simulink model "mass_model"  (R2023a)
settings: Solver=FixedStepAuto  StartTime=0.0  StopTime=10.0  FixedStep=0.4  RelTol=1e-3
libraries: simulink x2, rllib x1
settings Model: Creator=mori_keigo  LastModifiedBy=mori_keigo
settings OptimizationCC: ReuseModelBlockBuffer=off

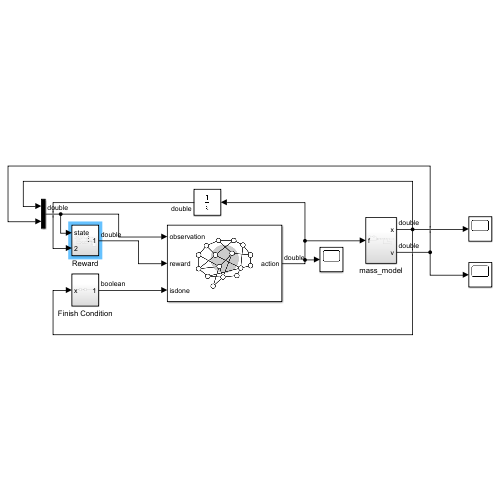
[thumbnail: Simulink's stored preview of the top-level diagram]
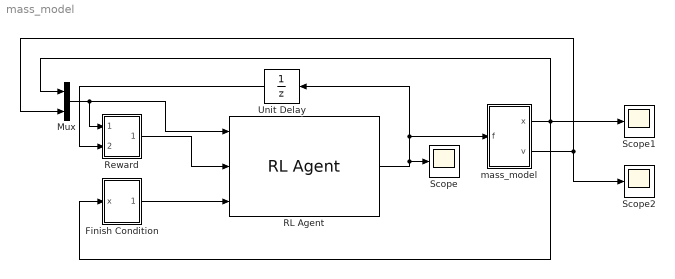
== system mass_model ==
  Finish Condition : Subsystem
  Mux : Mux  Inputs=2
  RL Agent : rllib/RL Agent  Agent=agentObj  ExternalActionAsInput=off  ProvideLastAction=off  ProvideCumRwd=off  TreatAsDirectFeedthrough=on  UseStrictObservationDataTypes=off
  Reward : Subsystem
  Scope : Scope
  Scope1 : Scope
  Scope2 : Scope
  Unit Delay : UnitDelay  SampleTime=-1  HasFrameUpgradeWarning=on
  mass_model : Subsystem
  wires:
  RL Agent/1 -> Unit Delay/1, mass_model/1(f), Scope/1
  mass_model/1(x) -> Scope1/1, Mux/1, Finish Condition/1(x)
  mass_model/2(v) -> Scope2/1, Mux/2
  Mux/1 -> Reward/1(state), RL Agent/1
  Reward/1(Out1) -> RL Agent/2
  Finish Condition/1(Out1) -> RL Agent/3
  Unit Delay/1 -> Reward/2(In2)

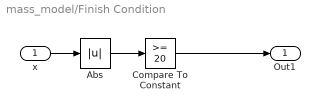
== system mass_model/Finish Condition ==
  x : Inport
  Abs : Abs  SaturateOnIntegerOverflow=off
  Compare To Constant : simulink/Logic and Bit Operations/Compare To Constant  relop=>=  const=20  OutDataTypeStr=boolean
  Out1 : Outport
  wires:
  Compare To Constant/1 -> Out1/1
  Abs/1 -> Compare To Constant/1
  x/1 -> Abs/1

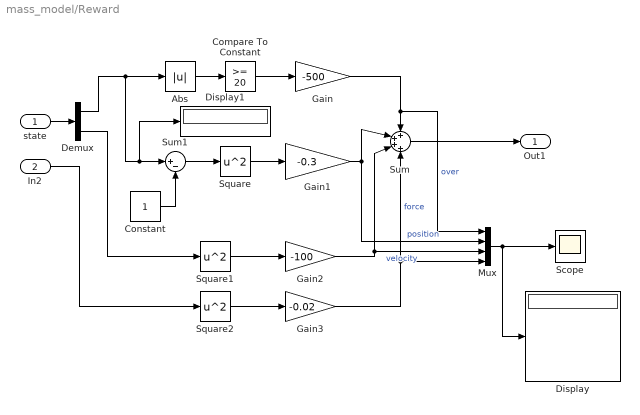
== system mass_model/Reward ==
  state : Inport
  In2 : Inport  Port=2
  Abs : Abs  SaturateOnIntegerOverflow=off
  Compare To Constant : simulink/Logic and Bit Operations/Compare To Constant  relop=>=  const=20  OutDataTypeStr=boolean
  Constant : Constant
  Demux : Demux  Outputs=2
  Display : Display
  Display1 : Display
  Gain : Gain  Gain=-500  OutDataTypeStr=double
  Gain1 : Gain  Gain=-0.3
  Gain2 : Gain  Gain=-100
  Gain3 : Gain  Gain=-0.02
  Mux : Mux
  Scope : Scope
  Square : Math  Operator=square
  Square1 : Math  Operator=square
  Square2 : Math  Operator=square
  Sum : Sum  Inputs=++++
  Sum1 : Sum  Inputs=|+-
  Out1 : Outport
  wires:
  state/1 -> Demux/1
  Demux/1 -> Display1/1, Sum1/1, Abs/1
  Abs/1 -> Compare To Constant/1
  Compare To Constant/1 -> Gain/1
  Square/1 -> Gain1/1
  Square1/1 -> Gain2/1
  Demux/2 -> Square1/1
  Gain/1 -> Mux/1, Sum/1  "over"
  Gain1/1 -> Mux/2, Sum/2  "position"
  Gain2/1 -> Mux/3, Sum/3  "velocity"
  Sum/1 -> Out1/1
  Constant/1 -> Sum1/2
  Sum1/1 -> Square/1
  In2/1 -> Square2/1
  Square2/1 -> Gain3/1
  Gain3/1 -> Mux/4, Sum/4  "force"
  Mux/1 -> Display/1, Scope/1

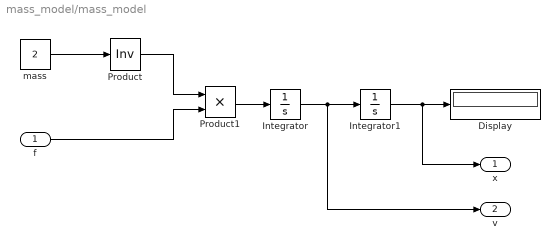
== system mass_model/mass_model ==
  f : Inport
  Display : Display
  Integrator : Integrator
  Integrator1 : Integrator
  Product : Product  Inputs=/  Multiplication=Matrix(*)
  Product1 : Product
  mass : Constant  Value=2
  x : Outport
  v : Outport  Port=2
  wires:
  mass/1 -> Product/1
  Integrator/1 -> v/1, Integrator1/1
  Integrator1/1 -> x/1, Display/1
  Product/1 -> Product1/1
  f/1 -> Product1/2
  Product1/1 -> Integrator/1
